simulink model "GaitGeneration"  (R2016b)
settings: Solver=VariableStepAuto  StartTime=0.0  StopTime=10.0  RelTol=1e-3
settings Model: Creator=march  LastModifiedBy=march

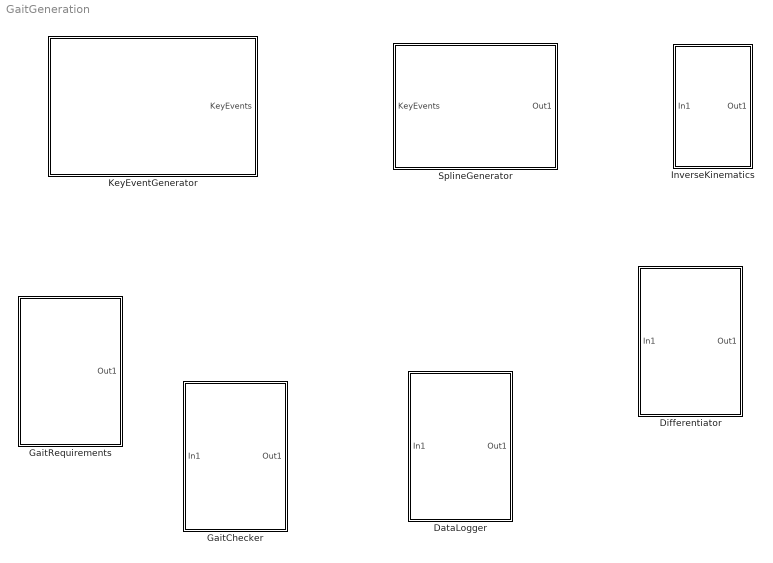
== system GaitGeneration ==
  DataLogger : Subsystem
  Differentiator : Subsystem
  GaitChecker : Subsystem
  GaitRequirements : Subsystem
  InverseKinematics : Subsystem
  KeyEventGenerator : Subsystem
  SplineGenerator : Subsystem

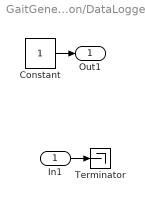
== system GaitGeneration/DataLogger ==
  In1 : Inport
  Constant : Constant
  Terminator : Terminator
  Out1 : Outport
  wires:
  In1/1 -> Terminator/1
  Constant/1 -> Out1/1

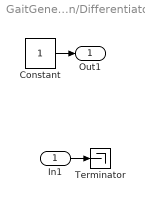
== system GaitGeneration/Differentiator ==
  In1 : Inport
  Constant : Constant
  Terminator : Terminator
  Out1 : Outport
  wires:
  In1/1 -> Terminator/1
  Constant/1 -> Out1/1

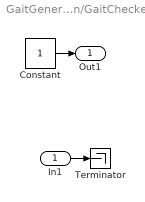
== system GaitGeneration/GaitChecker ==
  In1 : Inport
  Constant : Constant
  Terminator : Terminator
  Out1 : Outport
  wires:
  In1/1 -> Terminator/1
  Constant/1 -> Out1/1

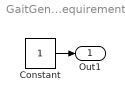
== system GaitGeneration/GaitRequirements ==
  Constant : Constant
  Out1 : Outport
  wires:
  Constant/1 -> Out1/1

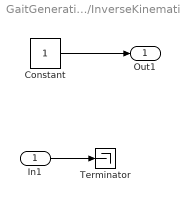
== system GaitGeneration/InverseKinematics ==
  In1 : Inport
  Constant : Constant
  Terminator : Terminator
  Out1 : Outport
  wires:
  Constant/1 -> Out1/1
  In1/1 -> Terminator/1

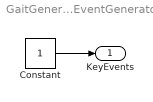
== system GaitGeneration/KeyEventGenerator ==
  Constant : Constant
  KeyEvents : Outport
  wires:
  Constant/1 -> KeyEvents/1

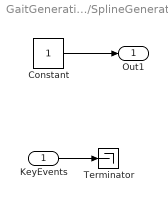
== system GaitGeneration/SplineGenerator ==
  KeyEvents : Inport
  Constant : Constant
  Terminator : Terminator
  Out1 : Outport
  wires:
  Constant/1 -> Out1/1
  KeyEvents/1 -> Terminator/1
